simulink subsystem "SD_2nd_Order_Modulator"  (R2020b)
settings: Solver=VariableStepAuto  StartTime=0.0  StopTime=10.0  RelTol=1e-3
settings Model: Creator=1111293  LastModifiedBy=1111293

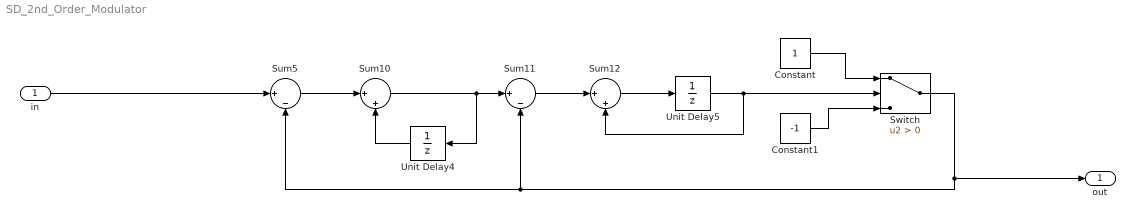
== system SD_2nd_Order_Modulator ==
  in : Inport
  Constant : Constant
  Constant1 : Constant  Value=-1
  Sum10 : Sum  Inputs=||+|+
  Sum11 : Sum  Inputs=||+|-
  Sum12 : Sum  Inputs=||+|+
  Sum5 : Sum  Inputs=||+|-
  Switch : Switch  Criteria=u2 > Threshold
  Unit Delay4 : UnitDelay  SampleTime=-1  HasFrameUpgradeWarning=on
  Unit Delay5 : UnitDelay  SampleTime=-1  HasFrameUpgradeWarning=on
  out : Outport
  wires:
  Constant/1 -> Switch/1
  Sum5/1 -> Sum10/1
  Unit Delay4/1 -> Sum10/2
  Sum10/1 -> Sum11/1, Unit Delay4/1
  Switch/1 -> Sum5/2, Sum11/2, out/1
  Sum11/1 -> Sum12/1
  Unit Delay5/1 -> Switch/2, Sum12/2
  Sum12/1 -> Unit Delay5/1
  Constant1/1 -> Switch/3
  in/1 -> Sum5/1
